simulink model "sim_regulation"  (R2022b)
settings: Solver=VariableStepAuto  StartTime=0.0  StopTime=T_SIM  MaxStep=0.001  RelTol=1e-3
undefined symbols (not defined in the file): control_par, controller_index, d, d_actual, omega_M, q_d, Q_INIT, r, r_actual
settings Model: Creator=alber  LastModifiedBy=alberto
settings OptimizationCC: ReuseModelBlockBuffer=on

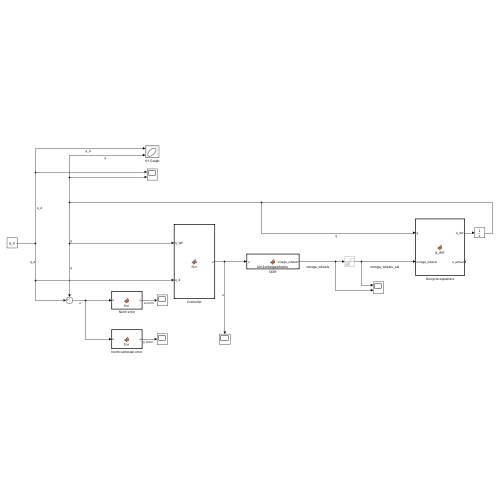
[thumbnail: Simulink's stored preview of the top-level diagram]
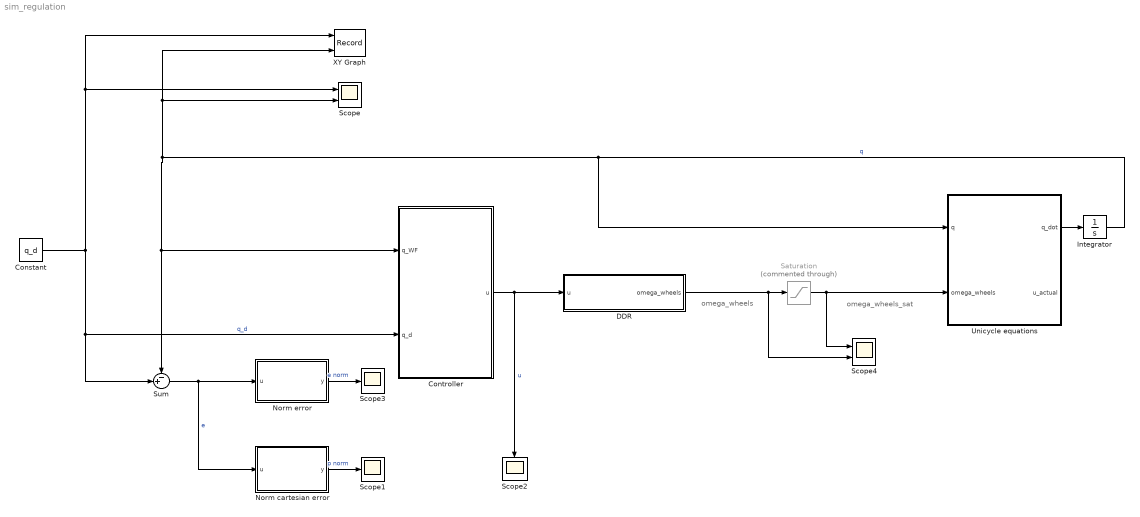
== system sim_regulation ==
  note: omega_wheels_sat
  note: omega_wheels
  Constant : Constant  Value=q_d
  Controller : MATLAB Function  TreatAsAtomicUnit=on
  DDR : MATLAB Function  TreatAsAtomicUnit=on
  Integrator : Integrator  InitialCondition=Q_INIT
  Norm cartesian error : MATLAB Function  TreatAsAtomicUnit=on
  Norm error : MATLAB Function  TreatAsAtomicUnit=on
  Saturation : Saturate  Commented=through  UpperLimit=omega_M  LowerLimit=-omega_M
  Scope : Scope  NumInputPorts=2
  Scope1 : Scope
  Scope2 : Scope
  Scope3 : Scope
  Scope4 : Scope  NumInputPorts=2
  Sum : Sum  Inputs=-+|
  Unicycle equations : MATLAB Function  TreatAsAtomicUnit=on
  XY Graph : Record  FileSettingsInternal="{\"entries\":[{\"content\":{\"excelSettings\":{\"content\":{},\"type\":\"Streamout.ExcelSettings\"}},\"type\":\"Streamout.FileSettingStorage\",\"uuid\":\"\"}],\"packageUris\":[\"http:\\/\\/schema.mathworks.com\\/mf0\\/streamout_blocks\\/R2020a\"],\"version\":\"1.0\"}"  Layout=[1 1]  SignalsInternal="{\"entries\":[{\"content\":{\"signals\":[{\"content\":{\"blockPath\":[],\"dimensions\":[3],\"domain\":\"\",\"hasChildren\":true,\"lineColor\":\"#ff6929\",\"port\":1,\"signalID\":5487,\"signalName\":\"q_d\"},\"type\":\"RecordBlkView.Signal\",\"uuid\":\"\"},{\"content\":{\"blockPath\":[],\"channel\":[1],\"dimensions\":[3],\"domain\":\"\",\"lineColor\":\"#d95319\",\"parentID\":5487,\"port\":1,\"signalID\":5488,\"signalName\":\"q_d\"},\"type\":\"RecordBlkView.Signal\",\"uuid\":\"\"},{\"content\":{\"blockPath\":[],\"channel\":[2],\"dimensions\":[3],\"domain\":\"\",\"lineColor\":\"#77ac30\",\"parentID\":5487,\"port\":1,\"signalID\":5489,\"signalName\":\"q_d\"},\"type\":\"RecordBlkView.Signal\",\"uuid\":\"\"},{\"content\":{\"blockPath\":[],\"channel\":[3],\"dimensions\":[3],\"domain\":\"\",\"lineColor\":\"#4dbeee\",\"parentID\":5487,\"port\":1,\"signalID\":5490,\"signalName\":\"q_d\"},\"type\":\"RecordBlkView.Signal\",\"uuid\":\"\"},{\"content\":{\"blockPath\":[],\"dimensions\":[3,1],\"domain\":\"\",\"hasChildren\":true,\"lineColor\":\"#a2142f\",\"port\":2,\"signalID\":5496,\"signalName\":\"q\"},\"type\":\"RecordBlkView.Signal\",\"uuid\":\"\"},{\"content\":{\"blockPath\":[],\"channel\":[1,1],\"dimensions\":[3,1],\"domain\":\"\",\"lineColor\":\"#000000\",\"lineStyle\":\"DASH_DOT\",\"parentID\":5496,\"plots\":[1],\"port\":2,\"signalID\":5497,\"signalName\":\"q\"},\"type\":\"RecordBlkView.Signal\",\"uuid\":\"\"},{\"content\":{\"blockPath\":[],\"channel\":[2,1],\"dimensions\":[3,1],\"domain\":\"\",\"lineColor\":\"#000000\",\"lineStyle\":\"DASH_DOT\",\"parentID\":5496,\"plots\":[1],\"port\":2,\"signalID\":5498,\"signalName\":\"q\"},\"type\":\"RecordBlkView.Signal\",\"uuid\":\"\"},{\"content\":{\"blockPath\":[],\"channel\":[3,1],\"dimensions\":[3,1],\"domain\":\"\",\"lineColor\":\"#b746ff\",\"parentID\":5496,\"port\":2,\"signalID\":5499,\"signalName\":\"q\"},\"type\":\"RecordBlkView.Signal\",\"uuid\":\"\"}]},\"type\":\"RecordBlkView.InputSignals\",\"uuid\":\"\"}],\"packageUris\":[\"http:\\/\\/schema.mathworks.com\\/mf0\\/streamout_blocks\\/R2020a\"],\"version\":\"1.0\"}"  VisualizationBindings="{\"xyplotplugin\":{\"info\":[{\"series\":[{\"bindingParametersList\":[{\"parameter\":\"X-Axis\",\"signalID\":5497,\"signalName\":\"q(1,1)\"},{\"parameter\":\"Y-Axis\",\"signalID\":5498,\"signalName\":\"q(2,1)\"}],\"seriesID\":25803}],\"subplotID\":1}]}}"  CompatibilityTag=XY
  wires:
  Integrator/1 -> Sum/1, Controller/1(q_WF), XY Graph/2, Scope/2, Unicycle equations/1(q)  "q"
  Unicycle equations/1(q_dot) -> Integrator/1
  Constant/1 -> Sum/2, Controller/2(q_d), XY Graph/1, Scope/1  "q_d"
  Sum/1 -> Norm cartesian error/1(u), Norm error/1(u)  "e"
  Controller/1(u) -> DDR/1(u), Scope2/1  "u"
  Norm cartesian error/1(y) -> Scope1/1  "p norm"
  DDR/1(omega_wheels) -> Saturation/1, Scope4/2
  Saturation/1 -> Unicycle equations/2(omega_wheels), Scope4/1
  Norm error/1(y) -> Scope3/1  "e norm"

== matlab function sim_regulation/Norm cartesian error ==
  data: u input; y output
function y = fcn(u)

y = sqrt(sum(u(1:2).^2));

== matlab function sim_regulation/Unicycle equations ==
  data: q input; omega_wheels input; q_dot output; r_actual parameter; d_actual parameter; u_actual output
function [q_dot, u_actual] = q_dot(q, omega_wheels, r_actual, d_actual)
u_actual = [r_actual/2, r_actual/2;-r_actual/d_actual, r_actual/d_actual]*omega_wheels;
theta = q(3);
q_dot = [[cos(theta), 0];[sin(theta), 0];[0,1]]*u_actual;

== matlab function sim_regulation/Norm error ==
  data: u input; y output
function y = fcn(u)
y = [u(1);u(2); wrapToPi(u(3))];

== matlab function sim_regulation/Controller ==
  data: q_WF input; q_d input; u output; controller_index parameter; control_par parameter
function u = fcn(q_WF, q_d, controller_index, control_par)
% select the controller
if controller_index == 1
    % cartesian regulator
    % transform q_WF
    % compute the input
    u = [0;0];
else
    % posture regulator
    % transform q_WF
    % compute pointing error
    u = [0;0];
end

== matlab function sim_regulation/DDR ==
  data: u input; omega_wheels output; r parameter; d parameter
function omega_wheels = kin2omegawheels(u, r, d)
omega_l = u(1)/r-d/(2*r)*u(2);
omega_r = u(1)/r+d/(2*r)*u(2);
omega_wheels = [omega_l;omega_r];
